simulink model "fullsystem"  (Simulink 8.5)
settings: Solver=ode15s  SolverMode=SingleTasking  StartTime=0.0  StopTime=0.1  RelTol=1e-3  AbsTol=1e-6
undefined symbols (not defined in the file or in its folder): DAB, den, elements, num
libraries: powerlib x43, powerlib_extras x1
(part 2 of 6)

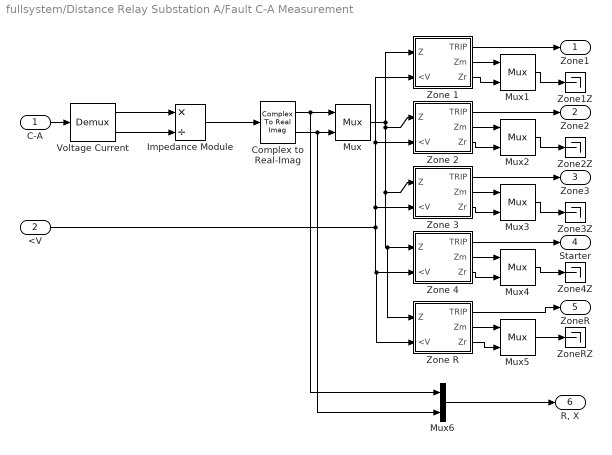
== system fullsystem/Distance Relay Substation A/Fault C-A Measurement ==
  C-A : Inport
  <V : Inport  Port=2
  Complex to Real-Imag : ComplexToRealImag
  Impedance Module : Product  Inputs=*/  SaturateOnIntegerOverflow=on  RndMeth=Zero  InputSameDT=on  OutDataTypeStr=Inherit: Same as first input
  Mux{,1..6} (7 alike) : Mux  Inputs=2
  Voltage Current : Demux  Outputs=2
  Zone 1 : Subsystem  mask(Zone){Xr=ZoneImpedance(1)*sin(LineAngle*pi/180), Rr=ZoneImpedance(1)*cos(LineAngle*pi/180), Td=ZoneTime(1)}
      mask prompts: Xr "Reactance reach [ohm]"; Rr "Resistance reach [ohm]"; Td "Time delay [s]"
  Zone 2 : Subsystem  mask(Zone){Xr=ZoneImpedance(2)*sin(LineAngle*pi/180), Rr=ZoneImpedance(2)*cos(LineAngle*pi/180), Td=ZoneTime(2)}
      mask prompts: Xr "Reactance reach [ohm]"; Rr "Resistance reach [ohm]"; Td "Time delay [s]"
  Zone 3 : Subsystem  mask(Zone){Xr=ZoneImpedance(3)*sin(LineAngle*pi/180), Rr=ZoneImpedance(3)*cos(LineAngle*pi/180), Td=ZoneTime(3)}
      mask prompts: Xr "Reactance reach [ohm]"; Rr "Resistance reach [ohm]"; Td "Time delay [s]"
  Zone 4 : Subsystem  mask(Zone){Xr=ZoneImpedance(4)*sin(LineAngle*pi/180), Rr=ZoneImpedance(4)*cos(LineAngle*pi/180), Td=ZoneTime(4)}
      mask prompts: Xr "Reactance reach [ohm]"; Rr "Resistance reach [ohm]"; Td "Time delay [s]"
  Zone R : Subsystem  mask(Zone){Xr=ZoneImpedance(5)*sin(LineAngle*pi/180), Rr=ZoneImpedance(5)*cos(LineAngle*pi/180), Td=ZoneTime(5)}
      mask prompts: Xr "Reactance reach [ohm]"; Rr "Resistance reach [ohm]"; Td "Time delay [s]"
  Zone1Z : Terminator
  Zone2Z : Terminator
  Zone3Z : Terminator
  Zone4Z : Terminator
  ZoneRZ : Terminator
  Zone1 : Outport  InitialOutput=0
  Zone2 : Outport  Port=2  InitialOutput=0
  Zone3 : Outport  Port=3  InitialOutput=0
  Starter : Outport  Port=4  InitialOutput=0
  ZoneR : Outport  Port=5  InitialOutput=0
  "R, X" : Outport  Port=6  InitialOutput=0
  wires:
  Voltage Current/2 -> Impedance Module/2
  Voltage Current/1 -> Impedance Module/1
  Impedance Module/1 -> Complex to Real-Imag/1
  Mux4/1 -> Zone4Z/1
  Mux3/1 -> Zone3Z/1
  Mux2/1 -> Zone2Z/1
  Mux1/1 -> Zone1Z/1
  <V/1 -> Zone R/2(<V), Zone 4/2(<V), Zone 3/2(<V), Zone 2/2(<V), Zone 1/2(<V)
  Complex to Real-Imag/2 -> Mux6/2, Mux/2
  Complex to Real-Imag/1 -> Mux6/1, Mux/1
  Zone 4/1(TRIP) -> Starter/1
  Zone 3/1(TRIP) -> Zone3/1
  Zone 2/1(TRIP) -> Zone2/1
  Zone 4/3(Zr) -> Mux4/2
  Zone 4/2(Zm) -> Mux4/1
  Zone 3/3(Zr) -> Mux3/2
  Zone 3/2(Zm) -> Mux3/1
  Zone 2/3(Zr) -> Mux2/2
  Zone 2/2(Zm) -> Mux2/1
  Zone 1/3(Zr) -> Mux1/2
  Zone 1/2(Zm) -> Mux1/1
  Zone 1/1(TRIP) -> Zone1/1
  Mux/1 -> Zone 2/1(Z), Zone R/1(Z), Zone 4/1(Z), Zone 3/1(Z), Zone 1/1(Z)
  C-A/1 -> Voltage Current/1
  Zone R/2(Zm) -> Mux5/1
  Zone R/3(Zr) -> Mux5/2
  Mux5/1 -> ZoneRZ/1
  Zone R/1(TRIP) -> ZoneR/1
  Mux6/1 -> "R, X"/1

== system fullsystem/Distance Relay Substation A/Fault C-G Measurement ==
  C-G : Inport
  <V : Inport  Port=2
  Complex to Real-Imag : ComplexToRealImag
  Impedance Module : Product  Inputs=*/  SaturateOnIntegerOverflow=on  RndMeth=Zero  InputSameDT=on  OutDataTypeStr=Inherit: Same as first input
  Mux{,1..6} (7 alike) : Mux  Inputs=2
  Voltage Current : Demux  Outputs=2
  Zone 1 : Subsystem  mask(Zone){Xr=ZoneImpedance(1)*sin(LineAngle*pi/180), Rr=ZoneImpedance(1)*cos(LineAngle*pi/180), Td=ZoneTime(1)}
      mask prompts: Xr "Reactance reach [ohm]"; Rr "Resistance reach [ohm]"; Td "Time delay [s]"
  Zone 2 : Subsystem  mask(Zone){Xr=ZoneImpedance(2)*sin(LineAngle*pi/180), Rr=ZoneImpedance(2)*cos(LineAngle*pi/180), Td=ZoneTime(2)}
      mask prompts: Xr "Reactance reach [ohm]"; Rr "Resistance reach [ohm]"; Td "Time delay [s]"
  Zone 3 : Subsystem  mask(Zone){Xr=ZoneImpedance(3)*sin(LineAngle*pi/180), Rr=ZoneImpedance(3)*cos(LineAngle*pi/180), Td=ZoneTime(3)}
      mask prompts: Xr "Reactance reach [ohm]"; Rr "Resistance reach [ohm]"; Td "Time delay [s]"
  Zone 4 : Subsystem  mask(Zone){Xr=ZoneImpedance(4)*sin(LineAngle*pi/180), Rr=ZoneImpedance(4)*cos(LineAngle*pi/180), Td=ZoneTime(4)}
      mask prompts: Xr "Reactance reach [ohm]"; Rr "Resistance reach [ohm]"; Td "Time delay [s]"
  Zone R : Subsystem  mask(Zone){Xr=ZoneImpedance(5)*sin(LineAngle*pi/180), Rr=ZoneImpedance(5)*cos(LineAngle*pi/180), Td=ZoneTime(5)}
      mask prompts: Xr "Reactance reach [ohm]"; Rr "Resistance reach [ohm]"; Td "Time delay [s]"
  Zone1Z : Terminator
  Zone2Z : Terminator
  Zone3Z : Terminator
  Zone4Z : Terminator
  ZoneRZ : Terminator
  Zone1 : Outport  InitialOutput=0
  Zone2 : Outport  Port=2  InitialOutput=0
  Zone3 : Outport  Port=3  InitialOutput=0
  Starter : Outport  Port=4  InitialOutput=0
  ZoneR : Outport  Port=5  InitialOutput=0
  "R, X" : Outport  Port=6  InitialOutput=0
  wires:
  Voltage Current/2 -> Impedance Module/2
  Voltage Current/1 -> Impedance Module/1
  Impedance Module/1 -> Complex to Real-Imag/1
  Mux4/1 -> Zone4Z/1
  Mux3/1 -> Zone3Z/1
  Mux2/1 -> Zone2Z/1
  Mux1/1 -> Zone1Z/1
  <V/1 -> Zone R/2(<V), Zone 4/2(<V), Zone 3/2(<V), Zone 2/2(<V), Zone 1/2(<V)
  Complex to Real-Imag/2 -> Mux6/2, Mux/2
  Complex to Real-Imag/1 -> Mux6/1, Mux/1
  Zone 4/1(TRIP) -> Starter/1
  Zone 3/1(TRIP) -> Zone3/1
  Zone 2/1(TRIP) -> Zone2/1
  Zone 4/3(Zr) -> Mux4/2
  Zone 4/2(Zm) -> Mux4/1
  Zone 3/3(Zr) -> Mux3/2
  Zone 3/2(Zm) -> Mux3/1
  Zone 2/3(Zr) -> Mux2/2
  Zone 2/2(Zm) -> Mux2/1
  Zone 1/3(Zr) -> Mux1/2
  Zone 1/2(Zm) -> Mux1/1
  Zone 1/1(TRIP) -> Zone1/1
  Mux/1 -> Zone 2/1(Z), Zone R/1(Z), Zone 4/1(Z), Zone 3/1(Z), Zone 1/1(Z)
  C-G/1 -> Voltage Current/1
  Zone R/2(Zm) -> Mux5/1
  Zone R/3(Zr) -> Mux5/2
  Mux5/1 -> ZoneRZ/1
  Zone R/1(TRIP) -> ZoneR/1
  Mux6/1 -> "R, X"/1

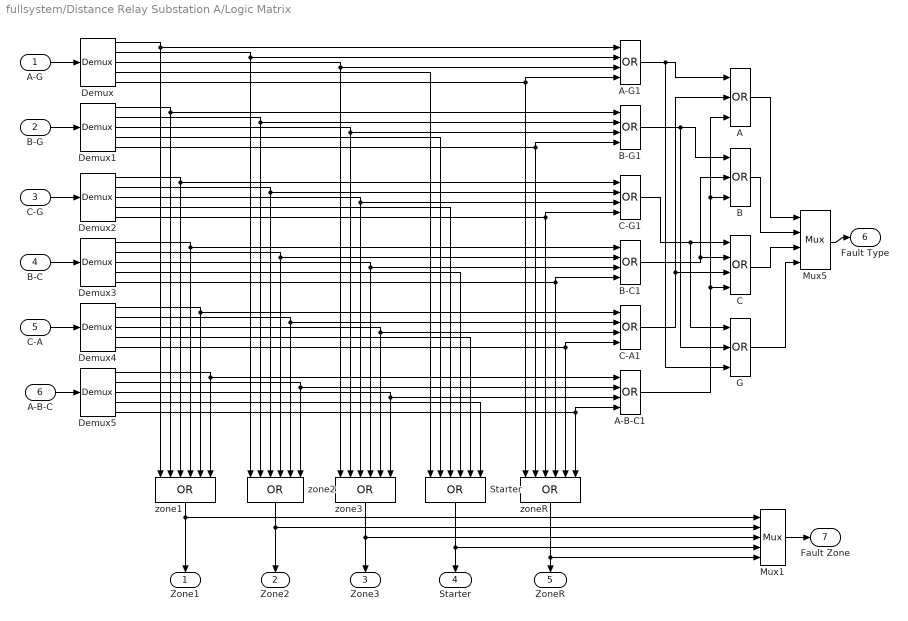
== system fullsystem/Distance Relay Substation A/Logic Matrix ==
  A-G : Inport
  B-G : Inport  Port=2
  C-G : Inport  Port=3
  B-C : Inport  Port=4
  C-A : Inport  Port=5
  A-B-C : Inport  Port=6
  A : Logic  Operator=OR  Inputs=3
  A-B-C1 : Logic  Operator=OR  Inputs=4
  "A-G1 " : Logic  Operator=OR  Inputs=4
  B : Logic  Operator=OR  Inputs=3
  B-C1 : Logic  Operator=OR  Inputs=4
  B-G1 : Logic  Operator=OR  Inputs=4
  C : Logic  Operator=OR  Inputs=4
  C-A1 : Logic  Operator=OR  Inputs=4
  C-G1 : Logic  Operator=OR  Inputs=4
  Demux{,1..5} (6 alike) : Demux  Outputs=5
  G : Logic  Operator=OR  Inputs=3
  Mux1 : Mux  Inputs=5
  Mux5 : Mux
  Starter : Logic  Operator=OR  Inputs=6
  zone1 : Logic  Operator=OR  Inputs=6
  zone2 : Logic  Operator=OR  Inputs=6
  zone3 : Logic  Operator=OR  Inputs=6
  zoneR : Logic  Operator=OR  Inputs=6
  " Zone1" : Outport  InitialOutput=0
  " Zone2" : Outport  Port=2  InitialOutput=0
  " Zone3" : Outport  Port=3  InitialOutput=0
  " Starter" : Outport  Port=4  InitialOutput=0
  " ZoneR" : Outport  Port=5  InitialOutput=0
  Fault Type : Outport  Port=6  InitialOutput=0
  Fault Zone : Outport  Port=7  InitialOutput=0
  wires:
  G/1 -> Mux5/4
  C/1 -> Mux5/3
  B/1 -> Mux5/2
  A/1 -> Mux5/1
  B-G1/1 -> G/2, B/1
  C-G1/1 -> G/1, C/1
  B-C1/1 -> C/2, B/2
  A-B-C1/1 -> B/3, A/3, C/4
  C-A1/1 -> A/2, C/3
  "A-G1 "/1 -> G/3, A/1
  A-G/1 -> Demux/1
  B-G/1 -> Demux1/1
  A-B-C/1 -> Demux5/1
  C-A/1 -> Demux4/1
  B-C/1 -> Demux3/1
  C-G/1 -> Demux2/1
  Mux5/1 -> Fault Type/1
  zone1/1 -> " Zone1"/1, Mux1/1
  zone2/1 -> Mux1/2, " Zone2"/1
  zoneR/1 -> Mux1/5, " ZoneR"/1
  zone3/1 -> " Zone3"/1, Mux1/3
  Starter/1 -> Mux1/4, " Starter"/1
  Mux1/1 -> Fault Zone/1
  Demux/5 -> zoneR/1, "A-G1 "/4
  Demux1/5 -> zoneR/2, B-G1/4
  Demux2/5 -> zoneR/3, C-G1/4
  Demux3/5 -> zoneR/4, B-C1/4
  Demux4/5 -> zoneR/5, C-A1/4
  Demux5/5 -> zoneR/6, A-B-C1/4
  Demux/1 -> "A-G1 "/1, zone1/1
  Demux1/1 -> B-G1/1, zone1/2
  Demux2/1 -> C-G1/1, zone1/3
  Demux3/1 -> B-C1/1, zone1/4
  Demux4/1 -> C-A1/1, zone1/5
  Demux5/1 -> A-B-C1/1, zone1/6
  Demux/2 -> "A-G1 "/2, zone2/1
  Demux1/2 -> B-G1/2, zone2/2
  Demux2/2 -> C-G1/2, zone2/3
  Demux3/2 -> B-C1/2, zone2/4
  Demux4/2 -> C-A1/2, zone2/5
  Demux5/2 -> A-B-C1/2, zone2/6
  Demux/3 -> "A-G1 "/3, zone3/1
  Demux1/3 -> B-G1/3, zone3/2
  Demux2/3 -> C-G1/3, zone3/3
  Demux3/3 -> B-C1/3, zone3/4
  Demux4/3 -> C-A1/3, zone3/5
  Demux5/3 -> A-B-C1/3, zone3/6
  Demux/4 -> Starter/1
  Demux1/4 -> Starter/2
  Demux2/4 -> Starter/3
  Demux3/4 -> Starter/4
  Demux4/4 -> Starter/5
  Demux5/4 -> Starter/6

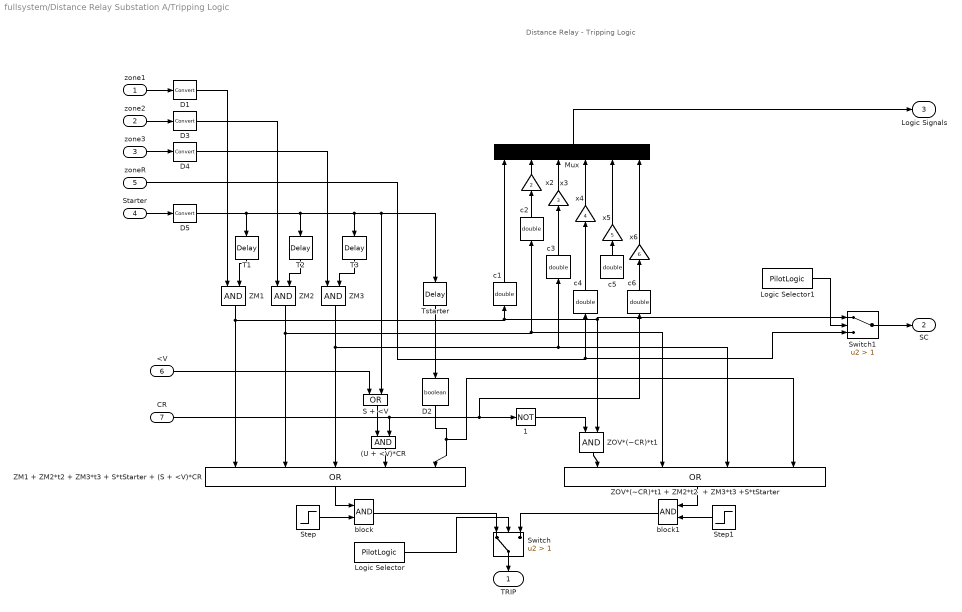
== system fullsystem/Distance Relay Substation A/Tripping Logic ==
  note: Distance Relay - Tripping Logic
  zone1 : Inport
  zone2 : Inport  Port=2
  zone3 : Inport  Port=3
  Starter : Inport  Port=4
  zoneR : Inport  Port=5
  <V : Inport  Port=6
  CR : Inport  Port=7
  (U + <V)*CR : Logic  AllPortsSameDT=off  OutDataTypeStr=boolean
  1 : Logic  Operator=NOT  AllPortsSameDT=off  OutDataTypeStr=boolean
  D{1,3..5} (4 alike) : DataTypeConversion
  D2 : DataTypeConversion  OutDataTypeStr=boolean
  Logic Selector : Constant  Value=PilotLogic  OutDataTypeStr=boolean
  Logic Selector1 : Constant  Value=PilotLogic  OutDataTypeStr=boolean
  Mux : Mux  Inputs=6
  S + <V : Logic  Operator=OR  AllPortsSameDT=off  OutDataTypeStr=boolean
  Step : Step  SampleTime=0
  Step1 : Step  SampleTime=0
  Switch : Switch  Criteria=u2 > Threshold  Threshold=1
  Switch1 : Switch  Criteria=u2 > Threshold  Threshold=1
  T1 : TransportDelay  DelayTime=ZoneTime(1)
  T2 : TransportDelay  DelayTime=ZoneTime(2)
  T3 : TransportDelay  DelayTime=ZoneTime(3)
  Tstarter : TransportDelay  DelayTime=Tstarter
  ZM1 : Logic  AllPortsSameDT=off  OutDataTypeStr=boolean
  ZM1 + ZM2*t2 + ZM3*t3 + S*tStarter + (S + <V)*CR : Logic  Operator=OR  Inputs=5
  ZM2 : Logic  AllPortsSameDT=off  OutDataTypeStr=boolean
  ZM3 : Logic  AllPortsSameDT=off  OutDataTypeStr=boolean
  ZOV*(~CR)*t1 : Logic  AllPortsSameDT=off  OutDataTypeStr=boolean
  ZOV*(~CR)*t1 + ZM2*t2  + ZM3*t3 +S*tStarter : Logic  Operator=OR  Inputs=4
  block : Logic  AllPortsSameDT=off  OutDataTypeStr=boolean
  block1 : Logic  AllPortsSameDT=off  OutDataTypeStr=boolean
  c{1..6} (6 alike) : DataTypeConversion  OutDataTypeStr=double
  x2 : Gain  Gain=2  SaturateOnIntegerOverflow=on  OutDataTypeStr=Inherit: Same as input  ParamDataTypeStr=Inherit: Same as input
  x3 : Gain  Gain=3  SaturateOnIntegerOverflow=on  OutDataTypeStr=Inherit: Same as input  ParamDataTypeStr=Inherit: Same as input
  x4 : Gain  Gain=4  SaturateOnIntegerOverflow=on  OutDataTypeStr=Inherit: Same as input  ParamDataTypeStr=Inherit: Same as input
  x5 : Gain  Gain=5  SaturateOnIntegerOverflow=on  OutDataTypeStr=Inherit: Same as input  ParamDataTypeStr=Inherit: Same as input
  x6 : Gain  Gain=6  SaturateOnIntegerOverflow=on  OutDataTypeStr=Inherit: Same as input  ParamDataTypeStr=Inherit: Same as input
  TRIP : Outport  InitialOutput=0
  SC : Outport  Port=2  InitialOutput=0
  Logic Signals : Outport  Port=3  InitialOutput=0
  wires:
  T1/1 -> ZM1/2
  T2/1 -> ZM2/2
  T3/1 -> ZM3/2
  ZM1/1 -> ZOV*(~CR)*t1/2, Switch1/1, c1/1, ZM1 + ZM2*t2 + ZM3*t3 + S*tStarter + (S + <V)*CR/1
  ZM2/1 -> c2/1, ZOV*(~CR)*t1 + ZM2*t2  + ZM3*t3 +S*tStarter/2, ZM1 + ZM2*t2 + ZM3*t3 + S*tStarter + (S + <V)*CR/2
  ZM3/1 -> c3/1, ZOV*(~CR)*t1 + ZM2*t2  + ZM3*t3 +S*tStarter/3, ZM1 + ZM2*t2 + ZM3*t3 + S*tStarter + (S + <V)*CR/3
  (U + <V)*CR/1 -> ZM1 + ZM2*t2 + ZM3*t3 + S*tStarter + (S + <V)*CR/4
  S + <V/1 -> (U + <V)*CR/1
  <V/1 -> S + <V/1
  x2/1 -> Mux/2
  x3/1 -> Mux/3
  x4/1 -> Mux/4
  x5/1 -> Mux/5
  x6/1 -> Mux/6
  Mux/1 -> Logic Signals/1
  ZOV*(~CR)*t1/1 -> ZOV*(~CR)*t1 + ZM2*t2  + ZM3*t3 +S*tStarter/1
  1/1 -> ZOV*(~CR)*t1/1
  ZM1 + ZM2*t2 + ZM3*t3 + S*tStarter + (S + <V)*CR/1 -> block/1
  Step/1 -> block/2
  Switch/1 -> TRIP/1
  Logic Selector/1 -> Switch/2
  block/1 -> Switch/1
  ZOV*(~CR)*t1 + ZM2*t2  + ZM3*t3 +S*tStarter/1 -> block1/1
  block1/1 -> Switch/3
  Step1/1 -> block1/2
  Switch1/1 -> SC/1
  Logic Selector1/1 -> Switch1/2
  zoneR/1 -> c4/1, Switch1/3
  c1/1 -> Mux/1
  c2/1 -> x2/1
  c3/1 -> x3/1
  c4/1 -> x4/1
  c5/1 -> x5/1
  c6/1 -> x6/1
  CR/1 -> 1/1, c6/1, (U + <V)*CR/2
  Tstarter/1 -> D2/1
  D2/1 -> ZOV*(~CR)*t1 + ZM2*t2  + ZM3*t3 +S*tStarter/4, ZM1 + ZM2*t2 + ZM3*t3 + S*tStarter + (S + <V)*CR/5
  zone1/1 -> D1/1
  D1/1 -> ZM1/1
  D3/1 -> ZM2/1
  zone2/1 -> D3/1
  zone3/1 -> D4/1
  D4/1 -> ZM3/1
  Starter/1 -> D5/1
  D5/1 -> T2/1, T3/1, Tstarter/1, S + <V/2, T1/1

== system fullsystem/Distance Relay Substation A/Undervoltage ==
  "Vabc  " : Inport
  Abs : Abs
  Abs1 : Abs
  Abs2 : Abs
  Demux2 : Demux  Outputs=3
  Logical Operator : Logic  Operator=OR  Inputs=3
  Relational Operator : RelationalOperator  Operator=<  InputSameDT=on
  Relational Operator1 : RelationalOperator  Operator=<  InputSameDT=on
  Relational Operator2 : RelationalOperator  Operator=<  InputSameDT=on
  underV  Threshold : Constant  Value=underV
  <V : Outport  InitialOutput=0
  wires:
  Demux2/3 -> Abs2/1
  Demux2/2 -> Abs1/1
  Abs1/1 -> Relational Operator2/1
  Abs2/1 -> Relational Operator1/1
  Demux2/1 -> Abs/1
  Abs/1 -> Relational Operator/1
  Relational Operator1/1 -> Logical Operator/3
  Relational Operator/1 -> Logical Operator/1
  Relational Operator2/1 -> Logical Operator/2
  Logical Operator/1 -> <V/1
  underV  Threshold/1 -> Relational Operator1/2, Relational Operator2/2, Relational Operator/2
  "Vabc  "/1 -> Demux2/1

== system fullsystem/Distance Relay Substation A1/Analog filtering, signal  conditioning ==
  note: Acquisition Block- analog filtering,
      | signal conditioning, sampling.
  Vin : Inport
  Iin : Inport  Port=2
  CURRENTS : Subsystem
  Mux{1..4} (4 alike) : Mux  Inputs=3
  VOLTAGES : Subsystem
  Vf : Outport  InitialOutput=0
  If : Outport  Port=2  InitialOutput=0
  If0 : Outport  Port=3  InitialOutput=0
  vf : Outport  Port=4  InitialOutput=0
  if : Outport  Port=5  InitialOutput=0
  wires:
  CURRENTS/4(k0I0f) -> If0/1
  Mux4/1 -> if/1
  Mux3/1 -> If/1
  CURRENTS/7(icf) -> Mux4/3
  CURRENTS/6(ibf) -> Mux4/2
  CURRENTS/5(iaf) -> Mux4/1
  CURRENTS/3(ICf) -> Mux3/3
  CURRENTS/2(IBf) -> Mux3/2
  CURRENTS/1(IAf) -> Mux3/1
  Iin/1 -> CURRENTS/1(Iabc)
  Mux2/1 -> vf/1
  VOLTAGES/6(vcf) -> Mux2/3
  VOLTAGES/5(vbf) -> Mux2/2
  VOLTAGES/4(vaf) -> Mux2/1
  VOLTAGES/3(VCf) -> Mux1/3
  VOLTAGES/2(VBf) -> Mux1/2
  VOLTAGES/1(VAf) -> Mux1/1
  Vin/1 -> VOLTAGES/1(Vabc)
  Mux1/1 -> Vf/1

== system fullsystem/Distance Relay Substation A1/Combination of Voltages  and Currents into 6 pairs  (for each type of fault) ==
  note: Voltage and current combination block
  Vf : Inport
  If : Inport  Port=2
  If0 : Inport  Port=3
  "Currents Ia, Ib, Ic, kIo" : Demux  Outputs=3
  Ia+kIo : Sum  SaturateOnIntegerOverflow=on  InputSameDT=on  OutDataTypeStr=Inherit: Same as first input
  Ia-Ib : Sum  Inputs=+-  SaturateOnIntegerOverflow=on  InputSameDT=on  OutDataTypeStr=Inherit: Same as first input
  Ib+kIo : Sum  SaturateOnIntegerOverflow=on  InputSameDT=on  OutDataTypeStr=Inherit: Same as first input
  Ib-Ic : Sum  Inputs=+-  SaturateOnIntegerOverflow=on  InputSameDT=on  OutDataTypeStr=Inherit: Same as first input
  Ic+kIo : Sum  SaturateOnIntegerOverflow=on  InputSameDT=on  OutDataTypeStr=Inherit: Same as first input
  Ic-Ia : Sum  Inputs=+-  SaturateOnIntegerOverflow=on  InputSameDT=on  OutDataTypeStr=Inherit: Same as first input
  Mux{10..15} (6 alike) : Mux  Inputs=2
  Va-Vb : Sum  Inputs=+-  SaturateOnIntegerOverflow=on  InputSameDT=on  OutDataTypeStr=Inherit: Same as first input
  Vb-Vc : Sum  Inputs=+-  SaturateOnIntegerOverflow=on  InputSameDT=on  OutDataTypeStr=Inherit: Same as first input
  Vc-Va : Sum  Inputs=+-  SaturateOnIntegerOverflow=on  InputSameDT=on  OutDataTypeStr=Inherit: Same as first input
  "Voltages Va,Vb, Vc" : Demux  Outputs=3
  "Volt, Curr A-G" : Outport  InitialOutput=0
  "Volt, Curr B-G" : Outport  Port=2  InitialOutput=0
  "Volt, Curr C-G" : Outport  Port=3  InitialOutput=0
  "Volt, Curr  B-C,B-C-G" : Outport  Port=4  InitialOutput=0
  "Volt, Curr C-A,C-A-G" : Outport  Port=5  InitialOutput=0
  "Volt, Curr A-B,A-B-C-G" : Outport  Port=6  InitialOutput=0
  wires:
  If0/1 -> Ib+kIo/2, Ia+kIo/2, Ic+kIo/2
  Mux13/1 -> "Volt, Curr  B-C,B-C-G"/1
  Vb-Vc/1 -> Mux13/1
  Ib-Ic/1 -> Mux13/2
  Mux12/1 -> "Volt, Curr C-G"/1
  Ic+kIo/1 -> Mux12/2
  If/1 -> "Currents Ia, Ib, Ic, kIo"/1
  "Voltages Va,Vb, Vc"/3 -> Vc-Va/1, Vb-Vc/2, Mux12/1
  "Voltages Va,Vb, Vc"/2 -> Vb-Vc/1, Mux11/1, Va-Vb/2
  "Voltages Va,Vb, Vc"/1 -> Va-Vb/1, Mux10/1, Vc-Va/2
  Vf/1 -> "Voltages Va,Vb, Vc"/1
  Mux15/1 -> "Volt, Curr A-B,A-B-C-G"/1
  Mux14/1 -> "Volt, Curr C-A,C-A-G"/1
  Vc-Va/1 -> Mux14/1
  Mux11/1 -> "Volt, Curr B-G"/1
  Mux10/1 -> "Volt, Curr A-G"/1
  Ia+kIo/1 -> Mux10/2
  Ib+kIo/1 -> Mux11/2
  Ic-Ia/1 -> Mux14/2
  Va-Vb/1 -> Mux15/1
  Ia-Ib/1 -> Mux15/2
  "Currents Ia, Ib, Ic, kIo"/2 -> Ia-Ib/2, Ib-Ic/1, Ib+kIo/1
  "Currents Ia, Ib, Ic, kIo"/3 -> Ic-Ia/1, Ib-Ic/2, Ic+kIo/1
  "Currents Ia, Ib, Ic, kIo"/1 -> Ia-Ib/1, Ic-Ia/2, Ia+kIo/1

== system fullsystem/Distance Relay Substation A1/Fault A-B-CMeasurement ==
  A-B-C : Inport
  <V : Inport  Port=2
  Complex to Real-Imag : ComplexToRealImag
  Impedance Module : Product  Inputs=*/  SaturateOnIntegerOverflow=on  RndMeth=Zero  InputSameDT=on  OutDataTypeStr=Inherit: Same as first input
  Mux{,1..6} (7 alike) : Mux  Inputs=2
  Voltage Current : Demux  Outputs=2
  Zone 1 : Subsystem  mask(Zone){Xr=ZoneImpedance(1)*sin(LineAngle*pi/180), Rr=ZoneImpedance(1)*cos(LineAngle*pi/180), Td=ZoneTime(1)}
      mask prompts: Xr "Reactance reach [ohm]"; Rr "Resistance reach [ohm]"; Td "Time delay [s]"
  Zone 2 : Subsystem  mask(Zone){Xr=ZoneImpedance(2)*sin(LineAngle*pi/180), Rr=ZoneImpedance(2)*cos(LineAngle*pi/180), Td=ZoneTime(2)}
      mask prompts: Xr "Reactance reach [ohm]"; Rr "Resistance reach [ohm]"; Td "Time delay [s]"
  Zone 3 : Subsystem  mask(Zone){Xr=ZoneImpedance(3)*sin(LineAngle*pi/180), Rr=ZoneImpedance(3)*cos(LineAngle*pi/180), Td=ZoneTime(3)}
      mask prompts: Xr "Reactance reach [ohm]"; Rr "Resistance reach [ohm]"; Td "Time delay [s]"
  Zone 4 : Subsystem  mask(Zone){Xr=ZoneImpedance(4)*sin(LineAngle*pi/180), Rr=ZoneImpedance(4)*cos(LineAngle*pi/180), Td=ZoneTime(4)}
      mask prompts: Xr "Reactance reach [ohm]"; Rr "Resistance reach [ohm]"; Td "Time delay [s]"
  Zone R : Subsystem  mask(Zone){Xr=ZoneImpedance(5)*sin(LineAngle*pi/180), Rr=ZoneImpedance(5)*cos(LineAngle*pi/180), Td=ZoneTime(5)}
      mask prompts: Xr "Reactance reach [ohm]"; Rr "Resistance reach [ohm]"; Td "Time delay [s]"
  Zone1Z : Terminator
  Zone2Z : Terminator
  Zone3Z : Terminator
  Zone4Z : Terminator
  ZoneRZ : Terminator
  Zone1 : Outport  InitialOutput=0
  Zone2 : Outport  Port=2  InitialOutput=0
  Zone3 : Outport  Port=3  InitialOutput=0
  Starter : Outport  Port=4  InitialOutput=0
  ZoneR : Outport  Port=5  InitialOutput=0
  "R, X" : Outport  Port=6  InitialOutput=0
  wires:
  Voltage Current/2 -> Impedance Module/2
  Voltage Current/1 -> Impedance Module/1
  Impedance Module/1 -> Complex to Real-Imag/1
  Mux4/1 -> Zone4Z/1
  Mux3/1 -> Zone3Z/1
  Mux2/1 -> Zone2Z/1
  Mux1/1 -> Zone1Z/1
  <V/1 -> Zone R/2(<V), Zone 4/2(<V), Zone 3/2(<V), Zone 2/2(<V), Zone 1/2(<V)
  Complex to Real-Imag/2 -> Mux6/2, Mux/2
  Complex to Real-Imag/1 -> Mux6/1, Mux/1
  Zone 4/1(TRIP) -> Starter/1
  Zone 3/1(TRIP) -> Zone3/1
  Zone 2/1(TRIP) -> Zone2/1
  Zone 4/3(Zr) -> Mux4/2
  Zone 4/2(Zm) -> Mux4/1
  Zone 3/3(Zr) -> Mux3/2
  Zone 3/2(Zm) -> Mux3/1
  Zone 2/3(Zr) -> Mux2/2
  Zone 2/2(Zm) -> Mux2/1
  Zone 1/3(Zr) -> Mux1/2
  Zone 1/2(Zm) -> Mux1/1
  Zone 1/1(TRIP) -> Zone1/1
  Mux/1 -> Zone 2/1(Z), Zone R/1(Z), Zone 4/1(Z), Zone 3/1(Z), Zone 1/1(Z)
  A-B-C/1 -> Voltage Current/1
  Zone R/2(Zm) -> Mux5/1
  Zone R/3(Zr) -> Mux5/2
  Mux5/1 -> ZoneRZ/1
  Zone R/1(TRIP) -> ZoneR/1
  Mux6/1 -> "R, X"/1

== system fullsystem/Distance Relay Substation A1/Fault A-G Measurement ==
  A-G : Inport
  <V : Inport  Port=2
  Complex to Real-Imag : ComplexToRealImag
  Impedance Module : Product  Inputs=*/  SaturateOnIntegerOverflow=on  RndMeth=Zero  InputSameDT=on  OutDataTypeStr=Inherit: Same as first input
  Mux{,1..6} (7 alike) : Mux  Inputs=2
  Voltage Current : Demux  Outputs=2
  Zone 1 : Subsystem  mask(Zone){Xr=ZoneImpedance(1)*sin(LineAngle*pi/180), Rr=ZoneImpedance(1)*cos(LineAngle*pi/180), Td=ZoneTime(1)}
      mask prompts: Xr "Reactance reach [ohm]"; Rr "Resistance reach [ohm]"; Td "Time delay [s]"
  Zone 2 : Subsystem  mask(Zone){Xr=ZoneImpedance(2)*sin(LineAngle*pi/180), Rr=ZoneImpedance(2)*cos(LineAngle*pi/180), Td=ZoneTime(2)}
      mask prompts: Xr "Reactance reach [ohm]"; Rr "Resistance reach [ohm]"; Td "Time delay [s]"
  Zone 3 : Subsystem  mask(Zone){Xr=ZoneImpedance(3)*sin(LineAngle*pi/180), Rr=ZoneImpedance(3)*cos(LineAngle*pi/180), Td=ZoneTime(3)}
      mask prompts: Xr "Reactance reach [ohm]"; Rr "Resistance reach [ohm]"; Td "Time delay [s]"
  Zone 4 : Subsystem  mask(Zone){Xr=ZoneImpedance(4)*sin(LineAngle*pi/180), Rr=ZoneImpedance(4)*cos(LineAngle*pi/180), Td=ZoneTime(4)}
      mask prompts: Xr "Reactance reach [ohm]"; Rr "Resistance reach [ohm]"; Td "Time delay [s]"
  Zone R : Subsystem  mask(Zone){Xr=ZoneImpedance(5)*sin(LineAngle*pi/180), Rr=ZoneImpedance(5)*cos(LineAngle*pi/180), Td=ZoneTime(5)}
      mask prompts: Xr "Reactance reach [ohm]"; Rr "Resistance reach [ohm]"; Td "Time delay [s]"
  Zone1Z : Terminator
  Zone2Z : Terminator
  Zone3Z : Terminator
  Zone4Z : Terminator
  ZoneRZ : Terminator
  Zone1 : Outport  InitialOutput=0
  Zone2 : Outport  Port=2  InitialOutput=0
  Zone3 : Outport  Port=3  InitialOutput=0
  Starter : Outport  Port=4  InitialOutput=0
  ZoneR : Outport  Port=5  InitialOutput=0
  "R, X" : Outport  Port=6  InitialOutput=0
  wires:
  Voltage Current/2 -> Impedance Module/2
  Voltage Current/1 -> Impedance Module/1
  Impedance Module/1 -> Complex to Real-Imag/1
  Mux4/1 -> Zone4Z/1
  Mux3/1 -> Zone3Z/1
  Mux2/1 -> Zone2Z/1
  Mux1/1 -> Zone1Z/1
  <V/1 -> Zone R/2(<V), Zone 4/2(<V), Zone 3/2(<V), Zone 2/2(<V), Zone 1/2(<V)
  Complex to Real-Imag/2 -> Mux6/2, Mux/2
  Complex to Real-Imag/1 -> Mux6/1, Mux/1
  Zone 4/1(TRIP) -> Starter/1
  Zone 3/1(TRIP) -> Zone3/1
  Zone 2/1(TRIP) -> Zone2/1
  Zone 4/3(Zr) -> Mux4/2
  Zone 4/2(Zm) -> Mux4/1
  Zone 3/3(Zr) -> Mux3/2
  Zone 3/2(Zm) -> Mux3/1
  Zone 2/3(Zr) -> Mux2/2
  Zone 2/2(Zm) -> Mux2/1
  Zone 1/3(Zr) -> Mux1/2
  Zone 1/2(Zm) -> Mux1/1
  Zone 1/1(TRIP) -> Zone1/1
  Mux/1 -> Zone 2/1(Z), Zone R/1(Z), Zone 4/1(Z), Zone 3/1(Z), Zone 1/1(Z)
  A-G/1 -> Voltage Current/1
  Zone R/2(Zm) -> Mux5/1
  Zone R/3(Zr) -> Mux5/2
  Mux5/1 -> ZoneRZ/1
  Zone R/1(TRIP) -> ZoneR/1
  Mux6/1 -> "R, X"/1

== system fullsystem/Distance Relay Substation A1/Fault B-C Measurement ==
  B-C : Inport
  <V : Inport  Port=2
  Complex to Real-Imag : ComplexToRealImag
  Impedance Module : Product  Inputs=*/  SaturateOnIntegerOverflow=on  RndMeth=Zero  InputSameDT=on  OutDataTypeStr=Inherit: Same as first input
  Mux{,1..6} (7 alike) : Mux  Inputs=2
  Voltage Current : Demux  Outputs=2
  Zone 1 : Subsystem  mask(Zone){Xr=ZoneImpedance(1)*sin(LineAngle*pi/180), Rr=ZoneImpedance(1)*cos(LineAngle*pi/180), Td=ZoneTime(1)}
      mask prompts: Xr "Reactance reach [ohm]"; Rr "Resistance reach [ohm]"; Td "Time delay [s]"
  Zone 2 : Subsystem  mask(Zone){Xr=ZoneImpedance(2)*sin(LineAngle*pi/180), Rr=ZoneImpedance(2)*cos(LineAngle*pi/180), Td=ZoneTime(2)}
      mask prompts: Xr "Reactance reach [ohm]"; Rr "Resistance reach [ohm]"; Td "Time delay [s]"
  Zone 3 : Subsystem  mask(Zone){Xr=ZoneImpedance(3)*sin(LineAngle*pi/180), Rr=ZoneImpedance(3)*cos(LineAngle*pi/180), Td=ZoneTime(3)}
      mask prompts: Xr "Reactance reach [ohm]"; Rr "Resistance reach [ohm]"; Td "Time delay [s]"
  Zone 4 : Subsystem  mask(Zone){Xr=ZoneImpedance(4)*sin(LineAngle*pi/180), Rr=ZoneImpedance(4)*cos(LineAngle*pi/180), Td=ZoneTime(4)}
      mask prompts: Xr "Reactance reach [ohm]"; Rr "Resistance reach [ohm]"; Td "Time delay [s]"
  Zone R : Subsystem  mask(Zone){Xr=ZoneImpedance(5)*sin(LineAngle*pi/180), Rr=ZoneImpedance(5)*cos(LineAngle*pi/180), Td=ZoneTime(5)}
      mask prompts: Xr "Reactance reach [ohm]"; Rr "Resistance reach [ohm]"; Td "Time delay [s]"
  Zone1Z : Terminator
  Zone2Z : Terminator
  Zone3Z : Terminator
  Zone4Z : Terminator
  ZoneRZ : Terminator
  Zone1 : Outport  InitialOutput=0
  Zone2 : Outport  Port=2  InitialOutput=0
  Zone3 : Outport  Port=3  InitialOutput=0
  Starter : Outport  Port=4  InitialOutput=0
  ZoneR : Outport  Port=5  InitialOutput=0
  "R, X" : Outport  Port=6  InitialOutput=0
  wires:
  Voltage Current/2 -> Impedance Module/2
  Voltage Current/1 -> Impedance Module/1
  Impedance Module/1 -> Complex to Real-Imag/1
  Mux4/1 -> Zone4Z/1
  Mux3/1 -> Zone3Z/1
  Mux2/1 -> Zone2Z/1
  Mux1/1 -> Zone1Z/1
  <V/1 -> Zone R/2(<V), Zone 4/2(<V), Zone 3/2(<V), Zone 2/2(<V), Zone 1/2(<V)
  Complex to Real-Imag/2 -> Mux6/2, Mux/2
  Complex to Real-Imag/1 -> Mux6/1, Mux/1
  Zone 4/1(TRIP) -> Starter/1
  Zone 3/1(TRIP) -> Zone3/1
  Zone 2/1(TRIP) -> Zone2/1
  Zone 4/3(Zr) -> Mux4/2
  Zone 4/2(Zm) -> Mux4/1
  Zone 3/3(Zr) -> Mux3/2
  Zone 3/2(Zm) -> Mux3/1
  Zone 2/3(Zr) -> Mux2/2
  Zone 2/2(Zm) -> Mux2/1
  Zone 1/3(Zr) -> Mux1/2
  Zone 1/2(Zm) -> Mux1/1
  Zone 1/1(TRIP) -> Zone1/1
  Mux/1 -> Zone 2/1(Z), Zone R/1(Z), Zone 4/1(Z), Zone 3/1(Z), Zone 1/1(Z)
  B-C/1 -> Voltage Current/1
  Zone R/2(Zm) -> Mux5/1
  Zone R/3(Zr) -> Mux5/2
  Mux5/1 -> ZoneRZ/1
  Zone R/1(TRIP) -> ZoneR/1
  Mux6/1 -> "R, X"/1

== system fullsystem/Distance Relay Substation A1/Fault B-G Measurement ==
  B-G : Inport
  <V : Inport  Port=2
  Complex to Real-Imag : ComplexToRealImag
  Impedance Module : Product  Inputs=*/  SaturateOnIntegerOverflow=on  RndMeth=Zero  InputSameDT=on  OutDataTypeStr=Inherit: Same as first input
  Mux{,1..6} (7 alike) : Mux  Inputs=2
  Voltage Current : Demux  Outputs=2
  Zone 1 : Subsystem  mask(Zone){Xr=ZoneImpedance(1)*sin(LineAngle*pi/180), Rr=ZoneImpedance(1)*cos(LineAngle*pi/180), Td=ZoneTime(1)}
      mask prompts: Xr "Reactance reach [ohm]"; Rr "Resistance reach [ohm]"; Td "Time delay [s]"
  Zone 2 : Subsystem  mask(Zone){Xr=ZoneImpedance(2)*sin(LineAngle*pi/180), Rr=ZoneImpedance(2)*cos(LineAngle*pi/180), Td=ZoneTime(2)}
      mask prompts: Xr "Reactance reach [ohm]"; Rr "Resistance reach [ohm]"; Td "Time delay [s]"
  Zone 3 : Subsystem  mask(Zone){Xr=ZoneImpedance(3)*sin(LineAngle*pi/180), Rr=ZoneImpedance(3)*cos(LineAngle*pi/180), Td=ZoneTime(3)}
      mask prompts: Xr "Reactance reach [ohm]"; Rr "Resistance reach [ohm]"; Td "Time delay [s]"
  Zone 4 : Subsystem  mask(Zone){Xr=ZoneImpedance(4)*sin(LineAngle*pi/180), Rr=ZoneImpedance(4)*cos(LineAngle*pi/180), Td=ZoneTime(4)}
      mask prompts: Xr "Reactance reach [ohm]"; Rr "Resistance reach [ohm]"; Td "Time delay [s]"
  Zone R : Subsystem  mask(Zone){Xr=ZoneImpedance(5)*sin(LineAngle*pi/180), Rr=ZoneImpedance(5)*cos(LineAngle*pi/180), Td=ZoneTime(5)}
      mask prompts: Xr "Reactance reach [ohm]"; Rr "Resistance reach [ohm]"; Td "Time delay [s]"
  Zone1Z : Terminator
  Zone2Z : Terminator
  Zone3Z : Terminator
  Zone4Z : Terminator
  ZoneRZ : Terminator
  Zone1 : Outport  InitialOutput=0
  Zone2 : Outport  Port=2  InitialOutput=0
  Zone3 : Outport  Port=3  InitialOutput=0
  Starter : Outport  Port=4  InitialOutput=0
  ZoneR : Outport  Port=5  InitialOutput=0
  "R, X" : Outport  Port=6  InitialOutput=0
  wires:
  Voltage Current/2 -> Impedance Module/2
  Voltage Current/1 -> Impedance Module/1
  Impedance Module/1 -> Complex to Real-Imag/1
  Mux4/1 -> Zone4Z/1
  Mux3/1 -> Zone3Z/1
  Mux2/1 -> Zone2Z/1
  Mux1/1 -> Zone1Z/1
  <V/1 -> Zone R/2(<V), Zone 4/2(<V), Zone 3/2(<V), Zone 2/2(<V), Zone 1/2(<V)
  Complex to Real-Imag/2 -> Mux6/2, Mux/2
  Complex to Real-Imag/1 -> Mux6/1, Mux/1
  Zone 4/1(TRIP) -> Starter/1
  Zone 3/1(TRIP) -> Zone3/1
  Zone 2/1(TRIP) -> Zone2/1
  Zone 4/3(Zr) -> Mux4/2
  Zone 4/2(Zm) -> Mux4/1
  Zone 3/3(Zr) -> Mux3/2
  Zone 3/2(Zm) -> Mux3/1
  Zone 2/3(Zr) -> Mux2/2
  Zone 2/2(Zm) -> Mux2/1
  Zone 1/3(Zr) -> Mux1/2
  Zone 1/2(Zm) -> Mux1/1
  Zone 1/1(TRIP) -> Zone1/1
  Mux/1 -> Zone 2/1(Z), Zone R/1(Z), Zone 4/1(Z), Zone 3/1(Z), Zone 1/1(Z)
  B-G/1 -> Voltage Current/1
  Zone R/2(Zm) -> Mux5/1
  Zone R/3(Zr) -> Mux5/2
  Mux5/1 -> ZoneRZ/1
  Zone R/1(TRIP) -> ZoneR/1
  Mux6/1 -> "R, X"/1

== system fullsystem/Distance Relay Substation A1/Fault C-A Measurement ==
  C-A : Inport
  <V : Inport  Port=2
  Complex to Real-Imag : ComplexToRealImag
  Impedance Module : Product  Inputs=*/  SaturateOnIntegerOverflow=on  RndMeth=Zero  InputSameDT=on  OutDataTypeStr=Inherit: Same as first input
  Mux{,1..6} (7 alike) : Mux  Inputs=2
  Voltage Current : Demux  Outputs=2
  Zone 1 : Subsystem  mask(Zone){Xr=ZoneImpedance(1)*sin(LineAngle*pi/180), Rr=ZoneImpedance(1)*cos(LineAngle*pi/180), Td=ZoneTime(1)}
      mask prompts: Xr "Reactance reach [ohm]"; Rr "Resistance reach [ohm]"; Td "Time delay [s]"
  Zone 2 : Subsystem  mask(Zone){Xr=ZoneImpedance(2)*sin(LineAngle*pi/180), Rr=ZoneImpedance(2)*cos(LineAngle*pi/180), Td=ZoneTime(2)}
      mask prompts: Xr "Reactance reach [ohm]"; Rr "Resistance reach [ohm]"; Td "Time delay [s]"
  Zone 3 : Subsystem  mask(Zone){Xr=ZoneImpedance(3)*sin(LineAngle*pi/180), Rr=ZoneImpedance(3)*cos(LineAngle*pi/180), Td=ZoneTime(3)}
      mask prompts: Xr "Reactance reach [ohm]"; Rr "Resistance reach [ohm]"; Td "Time delay [s]"
  Zone 4 : Subsystem  mask(Zone){Xr=ZoneImpedance(4)*sin(LineAngle*pi/180), Rr=ZoneImpedance(4)*cos(LineAngle*pi/180), Td=ZoneTime(4)}
      mask prompts: Xr "Reactance reach [ohm]"; Rr "Resistance reach [ohm]"; Td "Time delay [s]"
  Zone R : Subsystem  mask(Zone){Xr=ZoneImpedance(5)*sin(LineAngle*pi/180), Rr=ZoneImpedance(5)*cos(LineAngle*pi/180), Td=ZoneTime(5)}
      mask prompts: Xr "Reactance reach [ohm]"; Rr "Resistance reach [ohm]"; Td "Time delay [s]"
  Zone1Z : Terminator
  Zone2Z : Terminator
  Zone3Z : Terminator
  Zone4Z : Terminator
  ZoneRZ : Terminator
  Zone1 : Outport  InitialOutput=0
  Zone2 : Outport  Port=2  InitialOutput=0
  Zone3 : Outport  Port=3  InitialOutput=0
  Starter : Outport  Port=4  InitialOutput=0
  ZoneR : Outport  Port=5  InitialOutput=0
  "R, X" : Outport  Port=6  InitialOutput=0
  wires:
  Voltage Current/2 -> Impedance Module/2
  Voltage Current/1 -> Impedance Module/1
  Impedance Module/1 -> Complex to Real-Imag/1
  Mux4/1 -> Zone4Z/1
  Mux3/1 -> Zone3Z/1
  Mux2/1 -> Zone2Z/1
  Mux1/1 -> Zone1Z/1
  <V/1 -> Zone R/2(<V), Zone 4/2(<V), Zone 3/2(<V), Zone 2/2(<V), Zone 1/2(<V)
  Complex to Real-Imag/2 -> Mux6/2, Mux/2
  Complex to Real-Imag/1 -> Mux6/1, Mux/1
  Zone 4/1(TRIP) -> Starter/1
  Zone 3/1(TRIP) -> Zone3/1
  Zone 2/1(TRIP) -> Zone2/1
  Zone 4/3(Zr) -> Mux4/2
  Zone 4/2(Zm) -> Mux4/1
  Zone 3/3(Zr) -> Mux3/2
  Zone 3/2(Zm) -> Mux3/1
  Zone 2/3(Zr) -> Mux2/2
  Zone 2/2(Zm) -> Mux2/1
  Zone 1/3(Zr) -> Mux1/2
  Zone 1/2(Zm) -> Mux1/1
  Zone 1/1(TRIP) -> Zone1/1
  Mux/1 -> Zone 2/1(Z), Zone R/1(Z), Zone 4/1(Z), Zone 3/1(Z), Zone 1/1(Z)
  C-A/1 -> Voltage Current/1
  Zone R/2(Zm) -> Mux5/1
  Zone R/3(Zr) -> Mux5/2
  Mux5/1 -> ZoneRZ/1
  Zone R/1(TRIP) -> ZoneR/1
  Mux6/1 -> "R, X"/1

== system fullsystem/Distance Relay Substation A1/Fault C-G Measurement ==
  C-G : Inport
  <V : Inport  Port=2
  Complex to Real-Imag : ComplexToRealImag
  Impedance Module : Product  Inputs=*/  SaturateOnIntegerOverflow=on  RndMeth=Zero  InputSameDT=on  OutDataTypeStr=Inherit: Same as first input
  Mux{,1..6} (7 alike) : Mux  Inputs=2
  Voltage Current : Demux  Outputs=2
  Zone 1 : Subsystem  mask(Zone){Xr=ZoneImpedance(1)*sin(LineAngle*pi/180), Rr=ZoneImpedance(1)*cos(LineAngle*pi/180), Td=ZoneTime(1)}
      mask prompts: Xr "Reactance reach [ohm]"; Rr "Resistance reach [ohm]"; Td "Time delay [s]"
  Zone 2 : Subsystem  mask(Zone){Xr=ZoneImpedance(2)*sin(LineAngle*pi/180), Rr=ZoneImpedance(2)*cos(LineAngle*pi/180), Td=ZoneTime(2)}
      mask prompts: Xr "Reactance reach [ohm]"; Rr "Resistance reach [ohm]"; Td "Time delay [s]"
  Zone 3 : Subsystem  mask(Zone){Xr=ZoneImpedance(3)*sin(LineAngle*pi/180), Rr=ZoneImpedance(3)*cos(LineAngle*pi/180), Td=ZoneTime(3)}
      mask prompts: Xr "Reactance reach [ohm]"; Rr "Resistance reach [ohm]"; Td "Time delay [s]"
  Zone 4 : Subsystem  mask(Zone){Xr=ZoneImpedance(4)*sin(LineAngle*pi/180), Rr=ZoneImpedance(4)*cos(LineAngle*pi/180), Td=ZoneTime(4)}
      mask prompts: Xr "Reactance reach [ohm]"; Rr "Resistance reach [ohm]"; Td "Time delay [s]"
  Zone R : Subsystem  mask(Zone){Xr=ZoneImpedance(5)*sin(LineAngle*pi/180), Rr=ZoneImpedance(5)*cos(LineAngle*pi/180), Td=ZoneTime(5)}
      mask prompts: Xr "Reactance reach [ohm]"; Rr "Resistance reach [ohm]"; Td "Time delay [s]"
  Zone1Z : Terminator
  Zone2Z : Terminator
  Zone3Z : Terminator
  Zone4Z : Terminator
  ZoneRZ : Terminator
  Zone1 : Outport  InitialOutput=0
  Zone2 : Outport  Port=2  InitialOutput=0
  Zone3 : Outport  Port=3  InitialOutput=0
  Starter : Outport  Port=4  InitialOutput=0
  ZoneR : Outport  Port=5  InitialOutput=0
  "R, X" : Outport  Port=6  InitialOutput=0
  wires:
  Voltage Current/2 -> Impedance Module/2
  Voltage Current/1 -> Impedance Module/1
  Impedance Module/1 -> Complex to Real-Imag/1
  Mux4/1 -> Zone4Z/1
  Mux3/1 -> Zone3Z/1
  Mux2/1 -> Zone2Z/1
  Mux1/1 -> Zone1Z/1
  <V/1 -> Zone R/2(<V), Zone 4/2(<V), Zone 3/2(<V), Zone 2/2(<V), Zone 1/2(<V)
  Complex to Real-Imag/2 -> Mux6/2, Mux/2
  Complex to Real-Imag/1 -> Mux6/1, Mux/1
  Zone 4/1(TRIP) -> Starter/1
  Zone 3/1(TRIP) -> Zone3/1
  Zone 2/1(TRIP) -> Zone2/1
  Zone 4/3(Zr) -> Mux4/2
  Zone 4/2(Zm) -> Mux4/1
  Zone 3/3(Zr) -> Mux3/2
  Zone 3/2(Zm) -> Mux3/1
  Zone 2/3(Zr) -> Mux2/2
  Zone 2/2(Zm) -> Mux2/1
  Zone 1/3(Zr) -> Mux1/2
  Zone 1/2(Zm) -> Mux1/1
  Zone 1/1(TRIP) -> Zone1/1
  Mux/1 -> Zone 2/1(Z), Zone R/1(Z), Zone 4/1(Z), Zone 3/1(Z), Zone 1/1(Z)
  C-G/1 -> Voltage Current/1
  Zone R/2(Zm) -> Mux5/1
  Zone R/3(Zr) -> Mux5/2
  Mux5/1 -> ZoneRZ/1
  Zone R/1(TRIP) -> ZoneR/1
  Mux6/1 -> "R, X"/1

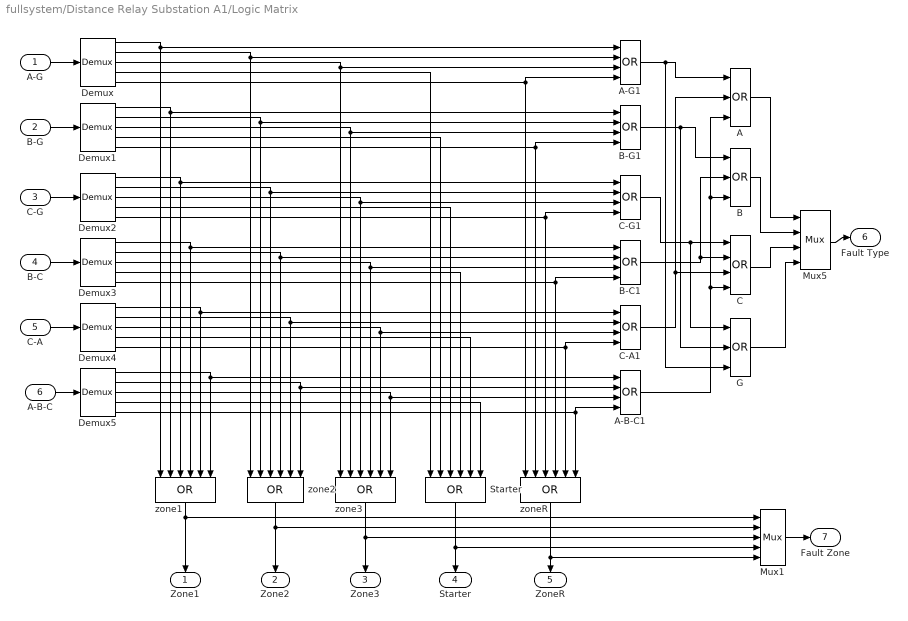
== system fullsystem/Distance Relay Substation A1/Logic Matrix ==
  A-G : Inport
  B-G : Inport  Port=2
  C-G : Inport  Port=3
  B-C : Inport  Port=4
  C-A : Inport  Port=5
  A-B-C : Inport  Port=6
  A : Logic  Operator=OR  Inputs=3
  A-B-C1 : Logic  Operator=OR  Inputs=4
  "A-G1 " : Logic  Operator=OR  Inputs=4
  B : Logic  Operator=OR  Inputs=3
  B-C1 : Logic  Operator=OR  Inputs=4
  B-G1 : Logic  Operator=OR  Inputs=4
  C : Logic  Operator=OR  Inputs=4
  C-A1 : Logic  Operator=OR  Inputs=4
  C-G1 : Logic  Operator=OR  Inputs=4
  Demux{,1..5} (6 alike) : Demux  Outputs=5
  G : Logic  Operator=OR  Inputs=3
  Mux1 : Mux  Inputs=5
  Mux5 : Mux
  Starter : Logic  Operator=OR  Inputs=6
  zone1 : Logic  Operator=OR  Inputs=6
  zone2 : Logic  Operator=OR  Inputs=6
  zone3 : Logic  Operator=OR  Inputs=6
  zoneR : Logic  Operator=OR  Inputs=6
  " Zone1" : Outport  InitialOutput=0
  " Zone2" : Outport  Port=2  InitialOutput=0
  " Zone3" : Outport  Port=3  InitialOutput=0
  " Starter" : Outport  Port=4  InitialOutput=0
  " ZoneR" : Outport  Port=5  InitialOutput=0
  Fault Type : Outport  Port=6  InitialOutput=0
  Fault Zone : Outport  Port=7  InitialOutput=0
  wires:
  G/1 -> Mux5/4
  C/1 -> Mux5/3
  B/1 -> Mux5/2
  A/1 -> Mux5/1
  B-G1/1 -> G/2, B/1
  C-G1/1 -> G/1, C/1
  B-C1/1 -> C/2, B/2
  A-B-C1/1 -> B/3, A/3, C/4
  C-A1/1 -> A/2, C/3
  "A-G1 "/1 -> G/3, A/1
  A-G/1 -> Demux/1
  B-G/1 -> Demux1/1
  A-B-C/1 -> Demux5/1
  C-A/1 -> Demux4/1
  B-C/1 -> Demux3/1
  C-G/1 -> Demux2/1
  Mux5/1 -> Fault Type/1
  zone1/1 -> " Zone1"/1, Mux1/1
  zone2/1 -> Mux1/2, " Zone2"/1
  zoneR/1 -> Mux1/5, " ZoneR"/1
  zone3/1 -> " Zone3"/1, Mux1/3
  Starter/1 -> Mux1/4, " Starter"/1
  Mux1/1 -> Fault Zone/1
  Demux/5 -> zoneR/1, "A-G1 "/4
  Demux1/5 -> zoneR/2, B-G1/4
  Demux2/5 -> zoneR/3, C-G1/4
  Demux3/5 -> zoneR/4, B-C1/4
  Demux4/5 -> zoneR/5, C-A1/4
  Demux5/5 -> zoneR/6, A-B-C1/4
  Demux/1 -> "A-G1 "/1, zone1/1
  Demux1/1 -> B-G1/1, zone1/2
  Demux2/1 -> C-G1/1, zone1/3
  Demux3/1 -> B-C1/1, zone1/4
  Demux4/1 -> C-A1/1, zone1/5
  Demux5/1 -> A-B-C1/1, zone1/6
  Demux/2 -> "A-G1 "/2, zone2/1
  Demux1/2 -> B-G1/2, zone2/2
  Demux2/2 -> C-G1/2, zone2/3
  Demux3/2 -> B-C1/2, zone2/4
  Demux4/2 -> C-A1/2, zone2/5
  Demux5/2 -> A-B-C1/2, zone2/6
  Demux/3 -> "A-G1 "/3, zone3/1
  Demux1/3 -> B-G1/3, zone3/2
  Demux2/3 -> C-G1/3, zone3/3
  Demux3/3 -> B-C1/3, zone3/4
  Demux4/3 -> C-A1/3, zone3/5
  Demux5/3 -> A-B-C1/3, zone3/6
  Demux/4 -> Starter/1
  Demux1/4 -> Starter/2
  Demux2/4 -> Starter/3
  Demux3/4 -> Starter/4
  Demux4/4 -> Starter/5
  Demux5/4 -> Starter/6

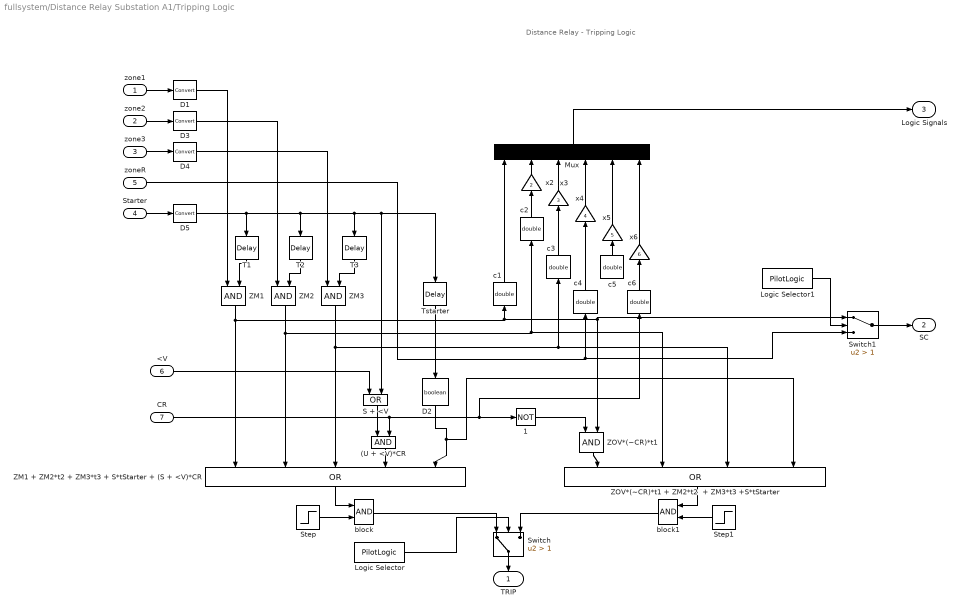
== system fullsystem/Distance Relay Substation A1/Tripping Logic ==
  note: Distance Relay - Tripping Logic
  zone1 : Inport
  zone2 : Inport  Port=2
  zone3 : Inport  Port=3
  Starter : Inport  Port=4
  zoneR : Inport  Port=5
  <V : Inport  Port=6
  CR : Inport  Port=7
  (U + <V)*CR : Logic  AllPortsSameDT=off  OutDataTypeStr=boolean
  1 : Logic  Operator=NOT  AllPortsSameDT=off  OutDataTypeStr=boolean
  D{1,3..5} (4 alike) : DataTypeConversion
  D2 : DataTypeConversion  OutDataTypeStr=boolean
  Logic Selector : Constant  Value=PilotLogic  OutDataTypeStr=boolean
  Logic Selector1 : Constant  Value=PilotLogic  OutDataTypeStr=boolean
  Mux : Mux  Inputs=6
  S + <V : Logic  Operator=OR  AllPortsSameDT=off  OutDataTypeStr=boolean
  Step : Step  SampleTime=0
  Step1 : Step  SampleTime=0
  Switch : Switch  Criteria=u2 > Threshold  Threshold=1
  Switch1 : Switch  Criteria=u2 > Threshold  Threshold=1
  T1 : TransportDelay  DelayTime=ZoneTime(1)
  T2 : TransportDelay  DelayTime=ZoneTime(2)
  T3 : TransportDelay  DelayTime=ZoneTime(3)
  Tstarter : TransportDelay  DelayTime=Tstarter
  ZM1 : Logic  AllPortsSameDT=off  OutDataTypeStr=boolean
  ZM1 + ZM2*t2 + ZM3*t3 + S*tStarter + (S + <V)*CR : Logic  Operator=OR  Inputs=5
  ZM2 : Logic  AllPortsSameDT=off  OutDataTypeStr=boolean
  ZM3 : Logic  AllPortsSameDT=off  OutDataTypeStr=boolean
  ZOV*(~CR)*t1 : Logic  AllPortsSameDT=off  OutDataTypeStr=boolean
  ZOV*(~CR)*t1 + ZM2*t2  + ZM3*t3 +S*tStarter : Logic  Operator=OR  Inputs=4
  block : Logic  AllPortsSameDT=off  OutDataTypeStr=boolean
  block1 : Logic  AllPortsSameDT=off  OutDataTypeStr=boolean
  c{1..6} (6 alike) : DataTypeConversion  OutDataTypeStr=double
  x2 : Gain  Gain=2  SaturateOnIntegerOverflow=on  OutDataTypeStr=Inherit: Same as input  ParamDataTypeStr=Inherit: Same as input
  x3 : Gain  Gain=3  SaturateOnIntegerOverflow=on  OutDataTypeStr=Inherit: Same as input  ParamDataTypeStr=Inherit: Same as input
  x4 : Gain  Gain=4  SaturateOnIntegerOverflow=on  OutDataTypeStr=Inherit: Same as input  ParamDataTypeStr=Inherit: Same as input
  x5 : Gain  Gain=5  SaturateOnIntegerOverflow=on  OutDataTypeStr=Inherit: Same as input  ParamDataTypeStr=Inherit: Same as input
  x6 : Gain  Gain=6  SaturateOnIntegerOverflow=on  OutDataTypeStr=Inherit: Same as input  ParamDataTypeStr=Inherit: Same as input
  TRIP : Outport  InitialOutput=0
  SC : Outport  Port=2  InitialOutput=0
  Logic Signals : Outport  Port=3  InitialOutput=0
  wires:
  T1/1 -> ZM1/2
  T2/1 -> ZM2/2
  T3/1 -> ZM3/2
  ZM1/1 -> ZOV*(~CR)*t1/2, Switch1/1, c1/1, ZM1 + ZM2*t2 + ZM3*t3 + S*tStarter + (S + <V)*CR/1
  ZM2/1 -> c2/1, ZOV*(~CR)*t1 + ZM2*t2  + ZM3*t3 +S*tStarter/2, ZM1 + ZM2*t2 + ZM3*t3 + S*tStarter + (S + <V)*CR/2
  ZM3/1 -> c3/1, ZOV*(~CR)*t1 + ZM2*t2  + ZM3*t3 +S*tStarter/3, ZM1 + ZM2*t2 + ZM3*t3 + S*tStarter + (S + <V)*CR/3
  (U + <V)*CR/1 -> ZM1 + ZM2*t2 + ZM3*t3 + S*tStarter + (S + <V)*CR/4
  S + <V/1 -> (U + <V)*CR/1
  <V/1 -> S + <V/1
  x2/1 -> Mux/2
  x3/1 -> Mux/3
  x4/1 -> Mux/4
  x5/1 -> Mux/5
  x6/1 -> Mux/6
  Mux/1 -> Logic Signals/1
  ZOV*(~CR)*t1/1 -> ZOV*(~CR)*t1 + ZM2*t2  + ZM3*t3 +S*tStarter/1
  1/1 -> ZOV*(~CR)*t1/1
  ZM1 + ZM2*t2 + ZM3*t3 + S*tStarter + (S + <V)*CR/1 -> block/1
  Step/1 -> block/2
  Switch/1 -> TRIP/1
  Logic Selector/1 -> Switch/2
  block/1 -> Switch/1
  ZOV*(~CR)*t1 + ZM2*t2  + ZM3*t3 +S*tStarter/1 -> block1/1
  block1/1 -> Switch/3
  Step1/1 -> block1/2
  Switch1/1 -> SC/1
  Logic Selector1/1 -> Switch1/2
  zoneR/1 -> c4/1, Switch1/3
  c1/1 -> Mux/1
  c2/1 -> x2/1
  c3/1 -> x3/1
  c4/1 -> x4/1
  c5/1 -> x5/1
  c6/1 -> x6/1
  CR/1 -> 1/1, c6/1, (U + <V)*CR/2
  Tstarter/1 -> D2/1
  D2/1 -> ZOV*(~CR)*t1 + ZM2*t2  + ZM3*t3 +S*tStarter/4, ZM1 + ZM2*t2 + ZM3*t3 + S*tStarter + (S + <V)*CR/5
  zone1/1 -> D1/1
  D1/1 -> ZM1/1
  D3/1 -> ZM2/1
  zone2/1 -> D3/1
  zone3/1 -> D4/1
  D4/1 -> ZM3/1
  Starter/1 -> D5/1
  D5/1 -> T2/1, T3/1, Tstarter/1, S + <V/2, T1/1

== system fullsystem/Distance Relay Substation A1/Undervoltage ==
  "Vabc  " : Inport
  Abs : Abs
  Abs1 : Abs
  Abs2 : Abs
  Demux2 : Demux  Outputs=3
  Logical Operator : Logic  Operator=OR  Inputs=3
  Relational Operator : RelationalOperator  Operator=<  InputSameDT=on
  Relational Operator1 : RelationalOperator  Operator=<  InputSameDT=on
  Relational Operator2 : RelationalOperator  Operator=<  InputSameDT=on
  underV  Threshold : Constant  Value=underV
  <V : Outport  InitialOutput=0
  wires:
  Demux2/3 -> Abs2/1
  Demux2/2 -> Abs1/1
  Abs1/1 -> Relational Operator2/1
  Abs2/1 -> Relational Operator1/1
  Demux2/1 -> Abs/1
  Abs/1 -> Relational Operator/1
  Relational Operator1/1 -> Logical Operator/3
  Relational Operator/1 -> Logical Operator/1
  Relational Operator2/1 -> Logical Operator/2
  Logical Operator/1 -> <V/1
  underV  Threshold/1 -> Relational Operator1/2, Relational Operator2/2, Relational Operator/2
  "Vabc  "/1 -> Demux2/1

== system fullsystem/Transsmision Line with fault (1, 2 or 3phase)/Fault Selector ==
  "  " : Constant  Value=faultType
  "  +" : Logic  Operator=OR
  " +" : Logic  Operator=OR  Inputs=4
  + : Logic  Operator=OR  Inputs=5
  "+ " : Logic  Operator=OR  Inputs=3
  A-B : Fcn  Expr=(u(1)==2)
  A-B-C : Fcn  Expr=(u(1)==4)
  A-B-C-G : Fcn  Expr=(u(1)==5)
  A-B-G : Fcn  Expr=(u(1)==3)
  A-G : Fcn  Expr=(u(1)==1)
  faultA : Outport  InitialOutput=0
  faultB : Outport  Port=2  InitialOutput=0
  faultC : Outport  Port=3  InitialOutput=0
  faultR : Outport  Port=4  InitialOutput=0
  wires:
  "  "/1 -> A-B-G/1, A-G/1, A-B/1, A-B-C-G/1, A-B-C/1
  +/1 -> faultA/1
  " +"/1 -> faultB/1
  "  +"/1 -> faultC/1
  "+ "/1 -> faultR/1
  A-B/1 -> +/2, " +"/1
  A-B-G/1 -> +/3, " +"/2, "+ "/2
  A-B-C/1 -> +/4, " +"/3, "  +"/1
  A-B-C-G/1 -> +/5, " +"/4, "  +"/2, "+ "/3
  A-G/1 -> +/1, "+ "/1

== system fullsystem/Transsmision Line with fault (1, 2 or 3phase)/Fault1 ==
  faultA : Inport
  faultB : Inport  Port=2
  faultC : Inport  Port=3
  faultG : Inport  Port=4
  Tfault : Inport  Port=5
  &{4..7} (4 alike) : Logic
  10000 ohms{1,3..5} (4 alike) : powerlib/Elements/Series RLC Branch  LConnTagsString=__new0  RConnTagsString=__new0  BranchType=R  Resistance=10000  Inductance=1e-3  SetiL0=off  InitialCurrent=0  Capacitance=1e-6  Setx0=off  InitialVoltage=0  Measurements=None
  Breaker3 : powerlib/Elements/Breaker  InitialState=0  SwitchingTimes="[ 1/60  5/60 ]"  External=on  BreakerResistance=0.01  SnubberResistance=1e6  SnubberCapacitance=inf  Measurements=None  MoreParameters=off  NoBreakLoop=off
  Breaker4 : powerlib/Elements/Breaker  InitialState=0  SwitchingTimes="[ 1/60  5/60 ]"  External=on  BreakerResistance=0.01  SnubberResistance=1e6  SnubberCapacitance=inf  Measurements=None  MoreParameters=off  NoBreakLoop=off
  Breaker5 : powerlib/Elements/Breaker  InitialState=0  SwitchingTimes="[ 1/60  5/60 ]"  External=on  BreakerResistance=0.01  SnubberResistance=1e6  SnubberCapacitance=inf  Measurements=None  MoreParameters=off  NoBreakLoop=off
  BreakerR1 : powerlib/Elements/Breaker  InitialState=0  SwitchingTimes="[ 1/60  5/60 ]"  External=on  BreakerResistance=0.01  SnubberResistance=1e6  SnubberCapacitance=inf  Measurements=None  MoreParameters=off  NoBreakLoop=off
  Ground1 : powerlib/Elements/Ground  LConnTagsString=a
  Rf A : powerlib/Elements/Series RLC Branch  LConnTagsString=__new0  RConnTagsString=__new0  BranchType=R  Resistance=faultR  Inductance=0  SetiL0=off  InitialCurrent=0  Capacitance=1e-6  Setx0=off  InitialVoltage=0  Measurements=None
  Rf B : powerlib/Elements/Series RLC Branch  LConnTagsString=__new0  RConnTagsString=__new0  BranchType=R  Resistance=faultR  Inductance=0  SetiL0=off  InitialCurrent=0  Capacitance=1e-6  Setx0=off  InitialVoltage=0  Measurements=None
  Rf C : powerlib/Elements/Series RLC Branch  LConnTagsString=__new0  RConnTagsString=__new0  BranchType=R  Resistance=faultR  Inductance=0  SetiL0=off  InitialCurrent=0  Capacitance=1e-6  Setx0=off  InitialVoltage=0  Measurements=None
  A : PMIOPort  Port=1  Side=Left
  B : PMIOPort  Port=2  Side=Left
  C : PMIOPort  Port=3  Side=Left
  wires:
  &6/1 -> Breaker5/1
  &5/1 -> Breaker4/1
  Tfault/1 -> &7/2, &6/2, &5/2, &4/2
  &7/1 -> BreakerR1/1
  faultG/1 -> &7/1
  faultC/1 -> &6/1
  faultB/1 -> &5/1
  faultA/1 -> &4/1
  &4/1 -> Breaker3/1
  connections:
  Rf B/RConn1 -- Rf C/RConn1 -- BreakerR1/LConn1 -- 10000 ohms1/LConn1 -- Rf A/RConn1
  BreakerR1/RConn1 -- 10000 ohms1/RConn1 -- Ground1/LConn1
  10000 ohms3/LConn1 -- A/RConn1 -- Breaker3/LConn1
  Rf A/LConn1 -- 10000 ohms3/RConn1 -- Breaker3/RConn1
  10000 ohms4/LConn1 -- B/RConn1 -- Breaker4/LConn1
  Rf B/LConn1 -- 10000 ohms4/RConn1 -- Breaker4/RConn1
  10000 ohms5/LConn1 -- C/RConn1 -- Breaker5/LConn1
  Rf C/LConn1 -- 10000 ohms5/RConn1 -- Breaker5/RConn1
